simulink model "2_4"  (R2017b)
settings: Solver=FixedStepAuto  StartTime=0.0  StopTime=5  FixedStep=1e-5  MaxStep=1e-4  RelTol=1e-3
libraries: powerlib x25
settings Model: NumberOfSteps=10  Creator=aniko  LastModifiedBy=aniko

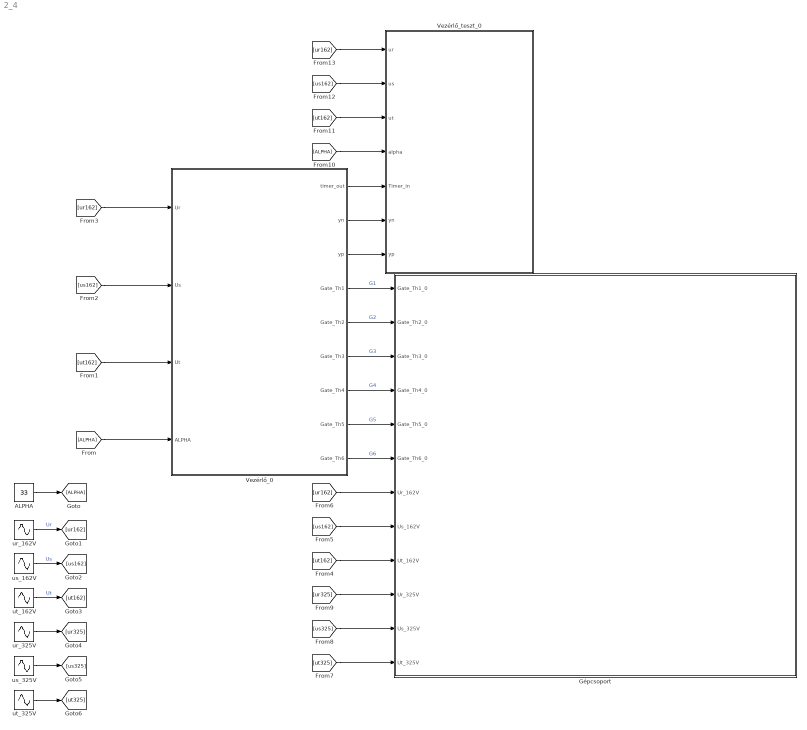
== system 2_4 ==
  "ALPHA " : Constant  Value=33
  "Gépcsoport " : Subsystem
  "Vezérlő_0 " : Subsystem
  Vezérlő_teszt_0 : Subsystem
  ur_162V : Sin  Amplitude=162  Frequency=50*2*pi  Phase=(2/3*pi)+(pi/2)  SampleTime=0
  "ur_325V " : Sin  Amplitude=325  Frequency=50*2*pi  Phase=(2/3*pi)  SampleTime=0
  us_162V : Sin  Amplitude=162  Frequency=50*2*pi  Phase=0+(pi/2)  SampleTime=0
  us_325V : Sin  Amplitude=325  Frequency=50*2*pi  SampleTime=0
  ut_162V : Sin  Amplitude=162  Frequency=50*2*pi  Phase=(4/3*pi)+(pi/2)  SampleTime=0
  ut_325V : Sin  Amplitude=325  Frequency=50*2*pi  Phase=(4/3)*pi  SampleTime=0
  wires:
  "Vezérlő_0 "/9("Gate_Th6 ") -> "Gépcsoport "/6(Gate_Th6_0)  "G6"
  "Vezérlő_0 "/8(Gate_Th5) -> "Gépcsoport "/5(Gate_Th5_0)  "G5"
  "Vezérlő_0 "/7("Gate_Th4 ") -> "Gépcsoport "/4(Gate_Th4_0)  "G4"
  "Vezérlő_0 "/6(Gate_Th3) -> "Gépcsoport "/3(Gate_Th3_0)  "G3"
  "Vezérlő_0 "/5("Gate_Th2 ") -> "Gépcsoport "/2(Gate_Th2_0)  "G2"
  "Vezérlő_0 "/4(Gate_Th1) -> "Gépcsoport "/1("Gate_Th1_0 ")  "G1"
  "ALPHA "/1 -> [ALPHA]
  ur_162V/1 -> [ur162]  "Ur"
  us_162V/1 -> [us162]  "Us"
  ut_162V/1 -> [ut162]  "Ut"
  "ur_325V "/1 -> [ur325]
  us_325V/1 -> [us325]
  ut_325V/1 -> [ut325]
  [ALPHA] -> "Vezérlő_0 "/4(ALPHA)
  [ut162] -> "Vezérlő_0 "/3(Ut)
  [us162] -> "Vezérlő_0 "/2(Us)
  [ur162] -> "Vezérlő_0 "/1(Ur)
  [ur162] -> "Gépcsoport "/7("Ur_162V ")
  [us162] -> "Gépcsoport "/8(Us_162V)
  [ut162] -> "Gépcsoport "/9(Ut_162V)
  [ur325] -> "Gépcsoport "/10(Ur_325V)
  [us325] -> "Gépcsoport "/11(Us_325V)
  [ut325] -> "Gépcsoport "/12("Ut_325V ")
  "Vezérlő_0 "/2(yn) -> Vezérlő_teszt_0/6("yn ")
  "Vezérlő_0 "/3("yp ") -> Vezérlő_teszt_0/7("yp ")
  "Vezérlő_0 "/1(timer_out) -> Vezérlő_teszt_0/5("Timer_in ")
  [ur162] -> Vezérlő_teszt_0/1(ur)
  [us162] -> Vezérlő_teszt_0/2(us)
  [ut162] -> Vezérlő_teszt_0/3("ut ")
  [ALPHA] -> Vezérlő_teszt_0/4("alpha ")

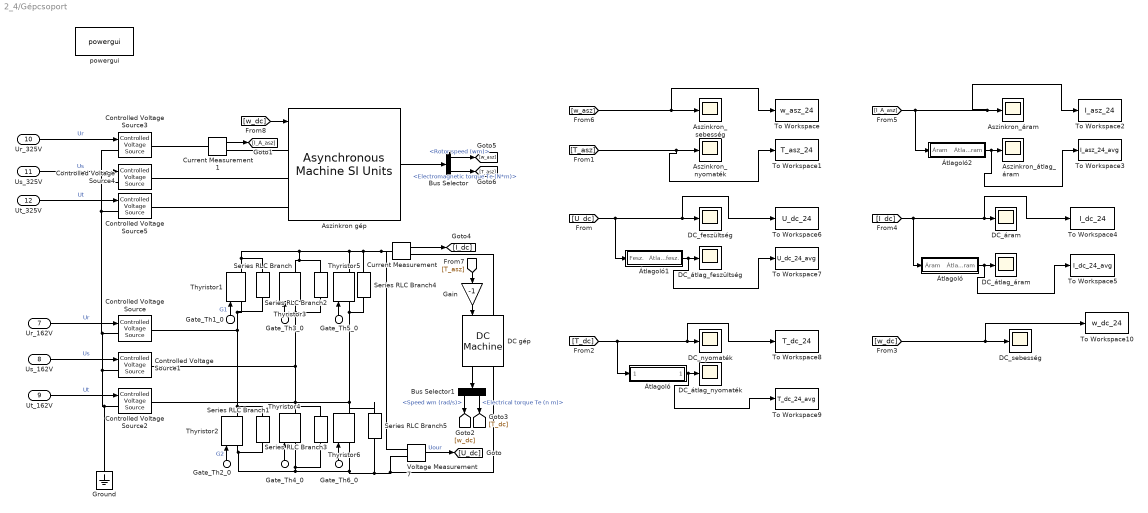
== system 2_4/Gépcsoport  ==
  "Gate_Th1_0 " : Inport
  Gate_Th2_0 : Inport  Port=2
  Gate_Th3_0 : Inport  Port=3
  Gate_Th4_0 : Inport  Port=4
  Gate_Th5_0 : Inport  Port=5
  Gate_Th6_0 : Inport  Port=6
  "Ur_162V " : Inport  Port=7
  Us_162V : Inport  Port=8
  Ut_162V : Inport  Port=9
  Ur_325V : Inport  Port=10
  Us_325V : Inport  Port=11
  "Ut_325V " : Inport  Port=12
  Aszinkron gép : powerlib/Machines/Asynchronous Machine SI Units  RotorType=Squirrel-cage  PresetModel=No  MechanicalLoad=Speed w  ShowDetailedParameters=on  ReferenceFrame=Rotor  Units=SI  MeasurementBus=off  NominalParameters=[5500 400 50]  Stator=[1 0.00565]  Rotor=[1 0.00565]  Cage1=[0.4155 0.002066]  Cage2=[0.4168 0.0003495]  Lm=0.091  Mechanical=[0.05 0.005879 3]  PolePairs=3  InitialConditions=[0 0 0 0 0 0 0 0]  SimulateSaturation=off  Saturation=[14.03593122, 27.81365428, 53.79336849, 72.68890987, 97.98006896, 148.6815601, 215.7428561, 302.9841135, 428.7778367 ; 230, 322, 414, 460, 506, 552, 598, 644, 690]  LoadFlowParameters=1492000  TsPowergui=0  TsBlock=-1  IterativeModel=Trapezoidal non iterative  IterativeDiscreteModel=Trapezoidal non iterative  Pmec=1.492e+006
  "Aszinkron_nyomaték " : Scope
  "Aszinkron_sebesség " : Scope
  Aszinkron_áram : Scope
  Aszinkron_átlag_áram : Scope
  Bus Selector : BusSelector  OutputSignals=Mechanical.Rotor speed (wm),Mechanical.Electromagnetic torque Te (N*m)
  Bus Selector1 : BusSelector  OutputSignals=Speed wm (rad/s),Electrical torque Te (n m)
  Controlled Voltage Source{,1..5} (6 alike) : powerlib/Electrical Sources/Controlled Voltage Source  Initialize=on  Source_Type=AC  Amplitude=0  Phase=0  Frequency=0  Measurements=None
  Current Measurement : powerlib/Measurements/Current Measurement  PhasorSimulation=off  OutputType=Complex  PSBequivalent=0
  Current Measurement1 : powerlib/Measurements/Current Measurement  PhasorSimulation=off  OutputType=Complex  PSBequivalent=0
  DC gép : powerlib/Machines/DC Machine  PresetModel=No  MechanicalLoad=Torque TL  FieldType=Permanent magnet  ShowDetailedParameters=on  MeasurementBus=off  RLa=[ 0.1 10e-3]  RLf="[ 240  120]"  Laf=1.8  MachineConstant=Back-emf constant (V/rpm)  Ke=205/1000  Kt=1.8  J=0.0325  Bm=0  Tf=0  w0=1  Ifinit=1  TsPowergui=0  TsBlock=-1
  "DC_feszültség " : Scope
  "DC_nyomaték " : Scope
  "DC_sebesség " : Scope
  "DC_áram " : Scope
  DC_átlag_feszültség : Scope
  "DC_átlag_nyomaték " : Scope
  DC_átlag_áram : Scope
  Gain : Gain  Gain=-1
  Ground : powerlib/Elements/Ground  LConnTagsString=a
  Series RLC Branch{,1..5} (6 alike) : powerlib/Elements/Series RLC Branch  LConnTagsString=__new0  RConnTagsString=__new0  BranchType=R  Resistance=100000  Inductance=1e-3  SetiL0=off  InitialCurrent=0  Capacitance=1e-6  Setx0=off  InitialVoltage=0  Measurements=None
  Thyristor{1..6} (6 alike) : powerlib/Power Electronics/Thyristor  Ron=0.001  Lon=0  Vf=0.8  IC=0  Rs=inf  Cs=250e-9  Measurements=on
  To Workspace : ToWorkspace  VariableName=w_asz_24  SaveFormat=Timeseries  SampleTime=-1
  To Workspace1 : ToWorkspace  VariableName=T_asz_24  SaveFormat=Timeseries  SampleTime=-1
  To Workspace10 : ToWorkspace  VariableName=w_dc_24  SaveFormat=Timeseries  SampleTime=-1
  To Workspace2 : ToWorkspace  VariableName=I_asz_24  SaveFormat=Timeseries  SampleTime=-1
  To Workspace3 : ToWorkspace  VariableName=I_asz_24_avg  SaveFormat=Timeseries  SampleTime=-1
  To Workspace4 : ToWorkspace  VariableName=I_dc_24  SaveFormat=Timeseries  SampleTime=-1
  To Workspace5 : ToWorkspace  VariableName=I_dc_24_avg  SaveFormat=Timeseries  SampleTime=-1
  To Workspace6 : ToWorkspace  VariableName=U_dc_24  SaveFormat=Timeseries  SampleTime=-1
  To Workspace7 : ToWorkspace  VariableName=U_dc_24_avg  SaveFormat=Timeseries  SampleTime=-1
  To Workspace8 : ToWorkspace  VariableName=T_dc_24  SaveFormat=Timeseries  SampleTime=-1
  To Workspace9 : ToWorkspace  VariableName=T_dc_24_avg  SaveFormat=Timeseries  SampleTime=-1
  Voltage Measurement7 : powerlib/Measurements/Voltage Measurement  PhasorSimulation=off  OutputType=Complex  PSBequivalent=0
  powergui : powerlib/powergui  Priority=1  SimulationMode=Discrete  SampleTime=1e-5  frequency=60  Iterations=50  frequencyindice=0  Pbase=100e6  ErrMax=1e-4  UnitsV=kV  UnitsW=MW  buscounter=0  FunctionMessages=off  echomessages=off  EnableUseOfTLC=off  CurrentSourceSwitches=off  DisableSnubberDevices=off  DisableRonSwitches=off  DisableVfSwitches=off  DisplayEquations=off  SolverType=Tustin/Backward Euler (TBE)  Interpol=off  ExternalGateDelay=off  methode=off  Ts=100  x0status=blocks  SPID=off  SwTol=0  HookPort=off  RestoreLinks=warning  ResistiveCurrentMeasurement=off  Frange=[0:2:500]  Ylog=off  Xlog=on  ShowGrid=off  save=off  variable=ZData  structure=0  ZoomFFT=off  StartTime=0.0  cycles=1  DisplayStyle=1  fundamental=60  FreqAxis=off  MaxFrequency=1000  frequencyindicesteady=1  RmsSteady=1  display=off
  Átlagoló : Subsystem
  "Átlagoló " : Subsystem
  Átlagoló1 : Subsystem
  Átlagoló2 : Subsystem
  wires:
  "Ur_162V "/1 -> Controlled Voltage Source/1  "Ur"
  Us_162V/1 -> Controlled Voltage Source1/1  "Us"
  Ut_162V/1 -> Controlled Voltage Source2/1  "Ut"
  Us_325V/1 -> Controlled Voltage Source4/1  "Us"
  Ur_325V/1 -> Controlled Voltage Source3/1  "Ur"
  "Ut_325V "/1 -> Controlled Voltage Source5/1  "Ut"
  "Gate_Th1_0 "/1 -> Thyristor1/1  "G1"
  Gate_Th3_0/1 -> Thyristor3/1
  Gate_Th4_0/1 -> Thyristor4/1
  Gate_Th5_0/1 -> Thyristor5/1
  Gate_Th6_0/1 -> Thyristor6/1
  Aszinkron gép/1 -> Bus Selector/1
  Voltage Measurement7/1 -> [U_dc]  "Uour"
  Gate_Th2_0/1 -> Thyristor2/1  "G2"
  Gain/1 -> DC gép/1
  Current Measurement1/1 -> [I_A_asz]
  [I_A_asz] -> Átlagoló2/1("Áram "), To Workspace2/1, Aszinkron_áram/1
  Átlagoló/1(Átlag_áram) -> To Workspace5/1, DC_átlag_áram/1
  DC gép/1 -> Bus Selector1/1
  Bus Selector1/1 -> [w_dc]  "<Speed wm (rad/s)>"
  Bus Selector1/2 -> [T_dc]  "<Electrical torque Te (n m)>"
  Átlagoló1/1(Átlag_fesz.) -> To Workspace7/1, DC_átlag_feszültség/1
  [T_dc] -> "Átlagoló "/1("Nyomaték "), To Workspace8/1, "DC_nyomaték "/1
  [w_dc] -> To Workspace10/1, "DC_sebesség "/1
  Current Measurement/1 -> [I_dc]
  [I_dc] -> Átlagoló/1("Áram "), To Workspace4/1, "DC_áram "/1
  Átlagoló2/1(Átlag_áram) -> To Workspace3/1, Aszinkron_átlag_áram/1
  Bus Selector/1 -> [w_asz]  "<Rotor speed (wm)>"
  Bus Selector/2 -> [T_asz]  "<Electromagnetic torque Te (N*m)>"
  [T_asz] -> To Workspace1/1, "Aszinkron_nyomaték "/1
  [w_asz] -> To Workspace/1, "Aszinkron_sebesség "/1
  [T_asz] -> Gain/1
  [w_dc] -> Aszinkron gép/1
  [U_dc] -> Átlagoló1/1("Fesz. "), To Workspace6/1, "DC_feszültség "/1
  "Átlagoló "/1(Átlag_nyomaték) -> To Workspace9/1, "DC_átlag_nyomaték "/1
  connections:
  Series RLC Branch/LConn1 -- Thyristor1/RConn1 -- Thyristor3/RConn1 -- Series RLC Branch2/LConn1 -- Thyristor5/RConn1 -- Current Measurement/LConn1 -- Voltage Measurement7/LConn1 -- Series RLC Branch4/LConn1
  Current Measurement1/LConn1 -- Controlled Voltage Source3/RConn1
  Aszinkron gép/LConn2 -- Controlled Voltage Source4/RConn1
  Aszinkron gép/LConn3 -- Controlled Voltage Source5/RConn1
  Controlled Voltage Source3/LConn1 -- Ground/LConn1 -- Controlled Voltage Source2/LConn1 -- Controlled Voltage Source1/LConn1 -- Controlled Voltage Source/LConn1 -- Controlled Voltage Source5/LConn1 -- Controlled Voltage Source4/LConn1
  Current Measurement1/RConn1 -- Aszinkron gép/LConn1
  Controlled Voltage Source/RConn1 -- Series RLC Branch1/LConn1 -- Thyristor2/RConn1 -- Series RLC Branch/RConn1 -- Thyristor1/LConn1
  Series RLC Branch2/RConn1 -- Thyristor3/LConn1 -- Series RLC Branch3/LConn1 -- Thyristor4/RConn1 -- Controlled Voltage Source1/RConn1
  Controlled Voltage Source2/RConn1 -- Series RLC Branch4/RConn1 -- Thyristor5/LConn1 -- Series RLC Branch5/LConn1 -- Thyristor6/RConn1
  Series RLC Branch1/RConn1 -- Thyristor2/LConn1 -- Thyristor4/LConn1 -- Series RLC Branch3/RConn1 -- DC gép/RConn1 -- Voltage Measurement7/LConn2 -- Series RLC Branch5/RConn1 -- Thyristor6/LConn1
  DC gép/LConn1 -- Current Measurement/RConn1

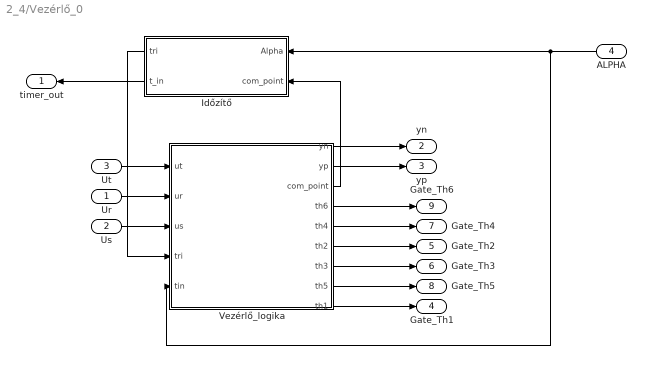
== system 2_4/Vezérlő_0  ==
  Ur : Inport
  Us : Inport  Port=2
  Ut : Inport  Port=3
  ALPHA : Inport  Port=4
  "Időzítő " : Subsystem  TreatAsAtomicUnit=on  SystemSampleTime=1e-5
      settings: MinAlgLoopOccurrences=on
  "Vezérlő_logika " : Stateflow chart  TreatAsAtomicUnit=on
  timer_out : Outport
  yn : Outport  Port=2
  "yp " : Outport  Port=3
  Gate_Th1 : Outport  Port=4
  "Gate_Th2 " : Outport  Port=5
  Gate_Th3 : Outport  Port=6
  "Gate_Th4 " : Outport  Port=7
  Gate_Th5 : Outport  Port=8
  "Gate_Th6 " : Outport  Port=9
  wires:
  Ur/1 -> "Vezérlő_logika "/2(ur)
  Us/1 -> "Vezérlő_logika "/3(us)
  "Vezérlő_logika "/1(yn) -> yn/1
  "Vezérlő_logika "/2(yp) -> "yp "/1
  Ut/1 -> "Vezérlő_logika "/1(ut)
  "Vezérlő_logika "/4(th6) -> "Gate_Th6 "/1
  "Vezérlő_logika "/8(th5) -> Gate_Th5/1
  "Időzítő "/2("t_in ") -> timer_out/1
  "Vezérlő_logika "/5(th4) -> "Gate_Th4 "/1
  "Vezérlő_logika "/7(th3) -> Gate_Th3/1
  "Vezérlő_logika "/9(th1) -> Gate_Th1/1
  "Vezérlő_logika "/6(th2) -> "Gate_Th2 "/1
  "Vezérlő_logika "/3(com_point) -> "Időzítő "/2(com_point)
  "Időzítő "/1(tri) -> "Vezérlő_logika "/4(tri)
  ALPHA/1 -> "Vezérlő_logika "/5(tin), "Időzítő "/1(Alpha)

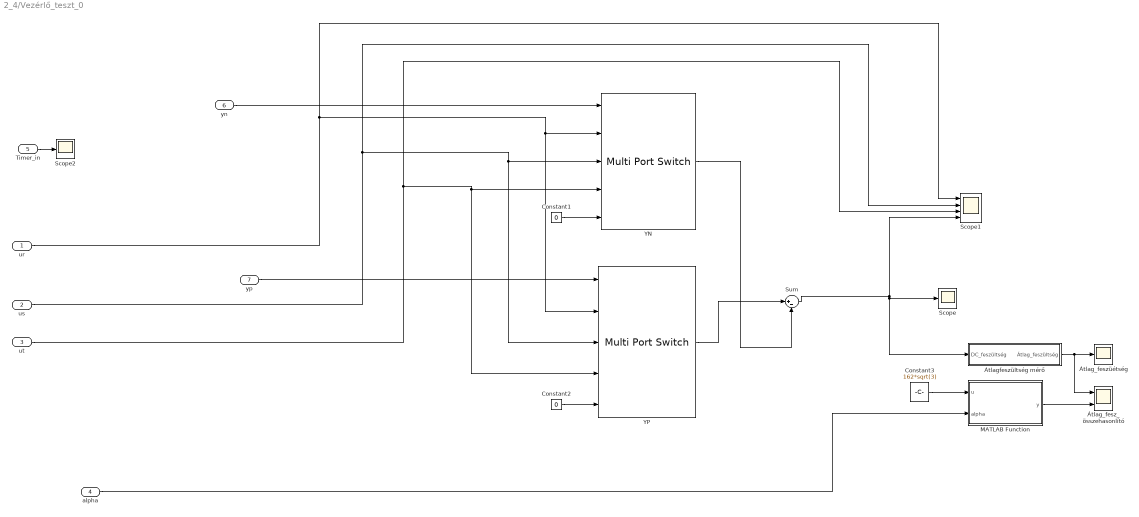
== system 2_4/Vezérlő_teszt_0 ==
  ur : Inport
  us : Inport  Port=2
  "ut " : Inport  Port=3
  "alpha " : Inport  Port=4
  "Timer_in " : Inport  Port=5
  "yn " : Inport  Port=6
  "yp " : Inport  Port=7
  Constant1 : Constant  Value=0
  Constant2 : Constant  Value=0
  Constant3 : Constant  Value=162*sqrt(3)
  MATLAB Function : MATLAB Function  TreatAsAtomicUnit=on
  Scope : Scope
  Scope1 : Scope  NumInputPorts=4
  Scope2 : Scope
  Sum : Sum  Inputs=|+-
  YN : MultiPortSwitch  Inputs=4
  "YP " : MultiPortSwitch  Inputs=4
  "Átlag_fesz_összehasonlító " : Scope  NumInputPorts=2
  "Átlag_feszüétség " : Scope
  Átlagfeszültség mérő : Subsystem
  wires:
  "yp "/1 -> "YP "/1
  "alpha "/1 -> MATLAB Function/2(alpha)
  us/1 -> Scope1/2, "YP "/3, YN/3
  Átlagfeszültség mérő/1("Átlag_feszültség ") -> "Átlag_fesz_összehasonlító "/1, "Átlag_feszüétség "/1
  ur/1 -> Scope1/1, "YP "/2, YN/2
  Constant3/1 -> MATLAB Function/1(u)
  "ut "/1 -> Scope1/3, "YP "/4, YN/4
  Sum/1 -> Scope/1, Átlagfeszültség mérő/1("DC_feszültség "), Scope1/4
  MATLAB Function/1(y) -> "Átlag_fesz_összehasonlító "/2
  Constant1/1 -> YN/5
  "yn "/1 -> YN/1
  Constant2/1 -> "YP "/5
  "Timer_in "/1 -> Scope2/1
  YN/1 -> Sum/2
  "YP "/1 -> Sum/1

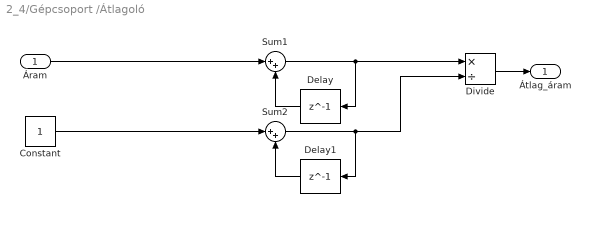
== system 2_4/Gépcsoport /Átlagoló ==
  "Áram " : Inport
  Constant : Constant  SampleTime=-1
  Delay : Delay  DelayLength=1  InitialCondition=0
  Delay1 : Delay  DelayLength=1  InitialCondition=0
  Divide : Product  Inputs=*/
  Sum1 : Sum  Inputs=|++
  Sum2 : Sum  Inputs=|++
  Átlag_áram : Outport
  wires:
  Sum1/1 -> Divide/1, Delay/1
  Delay/1 -> Sum1/2
  "Áram "/1 -> Sum1/1
  Sum2/1 -> Divide/2, Delay1/1
  Delay1/1 -> Sum2/2
  Constant/1 -> Sum2/1
  Divide/1 -> Átlag_áram/1

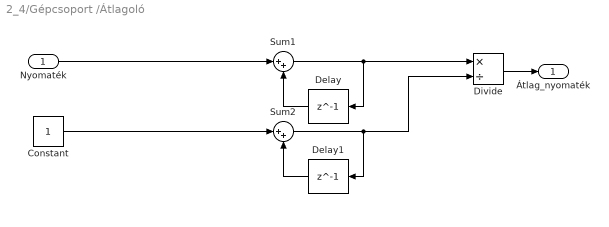
== system 2_4/Gépcsoport /Átlagoló  ==
  "Nyomaték " : Inport
  Constant : Constant  SampleTime=-1
  Delay : Delay  DelayLength=1  InitialCondition=0
  Delay1 : Delay  DelayLength=1  InitialCondition=0
  Divide : Product  Inputs=*/
  Sum1 : Sum  Inputs=|++
  Sum2 : Sum  Inputs=|++
  Átlag_nyomaték : Outport
  wires:
  Sum1/1 -> Divide/1, Delay/1
  Delay/1 -> Sum1/2
  "Nyomaték "/1 -> Sum1/1
  Sum2/1 -> Divide/2, Delay1/1
  Delay1/1 -> Sum2/2
  Constant/1 -> Sum2/1
  Divide/1 -> Átlag_nyomaték/1

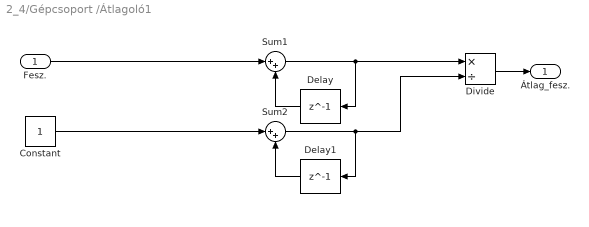
== system 2_4/Gépcsoport /Átlagoló1 ==
  "Fesz. " : Inport
  Constant : Constant  SampleTime=-1
  Delay : Delay  DelayLength=1  InitialCondition=0
  Delay1 : Delay  DelayLength=1  InitialCondition=0
  Divide : Product  Inputs=*/
  Sum1 : Sum  Inputs=|++
  Sum2 : Sum  Inputs=|++
  Átlag_fesz. : Outport
  wires:
  Sum1/1 -> Divide/1, Delay/1
  Delay/1 -> Sum1/2
  "Fesz. "/1 -> Sum1/1
  Sum2/1 -> Divide/2, Delay1/1
  Delay1/1 -> Sum2/2
  Constant/1 -> Sum2/1
  Divide/1 -> Átlag_fesz./1

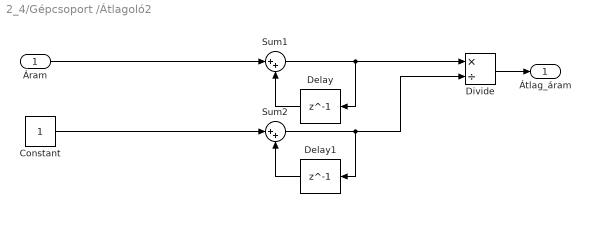
== system 2_4/Gépcsoport /Átlagoló2 ==
  "Áram " : Inport
  Constant : Constant  SampleTime=-1
  Delay : Delay  DelayLength=1  InitialCondition=0
  Delay1 : Delay  DelayLength=1  InitialCondition=0
  Divide : Product  Inputs=*/
  Sum1 : Sum  Inputs=|++
  Sum2 : Sum  Inputs=|++
  Átlag_áram : Outport
  wires:
  Sum1/1 -> Divide/1, Delay/1
  Delay/1 -> Sum1/2
  "Áram "/1 -> Sum1/1
  Sum2/1 -> Divide/2, Delay1/1
  Delay1/1 -> Sum2/2
  Constant/1 -> Sum2/1
  Divide/1 -> Átlag_áram/1

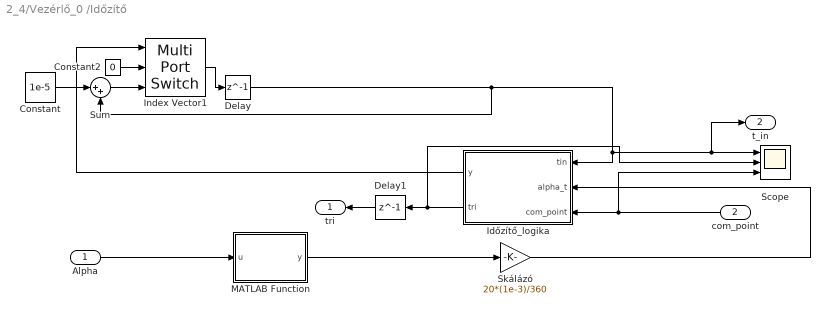
== system 2_4/Vezérlő_0 /Időzítő  ==
  Alpha : Inport
  com_point : Inport  Port=2
  Constant : Constant  Value=1e-5  SampleTime=-1
  Constant2 : Constant  Value=0
  Delay : Delay  DelayLength=1  InitialCondition=0
  Delay1 : Delay  DelayLength=1  InitialCondition=0
  "Időzítő_logika " : Stateflow chart  TreatAsAtomicUnit=on
  Index Vector1 : MultiPortSwitch  DataPortOrder=Zero-based contiguous  Inputs=2  zeroidx=on
  MATLAB Function : MATLAB Function  TreatAsAtomicUnit=on
  Scope : Scope  NumInputPorts=3
  Skálázó : Gain  Gain=20*(1e-3)/360
  Sum : Sum  Inputs=|++
  tri : Outport
  "t_in " : Outport  Port=2
  wires:
  Sum/1 -> Index Vector1/3
  Constant/1 -> Sum/1
  "Időzítő_logika "/1(y) -> Index Vector1/1
  Skálázó/1 -> "Időzítő_logika "/2(alpha_t)
  com_point/1 -> Scope/3, "Időzítő_logika "/3(com_point)
  "Időzítő_logika "/2(tri) -> Delay1/1, Scope/2
  Delay/1 -> "Időzítő_logika "/1(tin), "t_in "/1, Scope/1, Sum/2
  Constant2/1 -> Index Vector1/2
  Index Vector1/1 -> Delay/1
  Delay1/1 -> tri/1
  MATLAB Function/1(y) -> Skálázó/1
  Alpha/1 -> MATLAB Function/1(u)

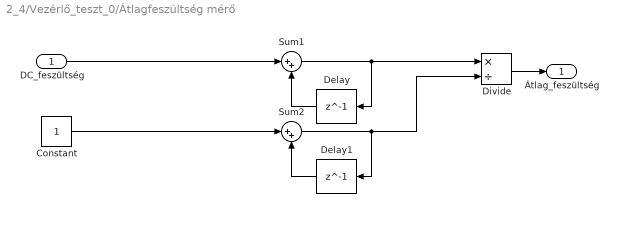
== system 2_4/Vezérlő_teszt_0/Átlagfeszültség mérő ==
  "DC_feszültség " : Inport
  Constant : Constant  SampleTime=-1
  Delay : Delay  DelayLength=1  InitialCondition=0
  Delay1 : Delay  DelayLength=1  InitialCondition=0
  Divide : Product  Inputs=*/
  Sum1 : Sum  Inputs=|++
  Sum2 : Sum  Inputs=|++
  "Átlag_feszültség " : Outport
  wires:
  Sum1/1 -> Divide/1, Delay/1
  Delay/1 -> Sum1/2
  "DC_feszültség "/1 -> Sum1/1
  Sum2/1 -> Divide/2, Delay1/1
  Delay1/1 -> Sum2/2
  Constant/1 -> Sum2/1
  Divide/1 -> "Átlag_feszültség "/1

== matlab function 2_4/Vezérlő_teszt_0/MATLAB Function ==
  data: u input; y output; alpha input
function y =aramiranyito(u, alpha)

%Az áramirányító elméleti kimeneti feszültsége.

y=u*(3/pi)*cos((alpha*(2*pi)/360));

== matlab function 2_4/Vezérlő_0 /Időzítő /MATLAB Function ==
  data: u input; y output
function y =idozito(u)
%Az időzítő helyes beállítására szolgál.


if u<=0,
 y=0;
elseif u>0 && u<60,
 y=u;
elseif u>=60 && u<120,
 y=u-60;    
elseif u>=120 && u<180,
 y=u-120;
else
 y=59;
end;

== stateflow chart 2_4/Vezérlő_0 /Időzítő /Időzítő_logika  ==
  state RESET
    during: y=0;
    tri=0;
  state COUNTING
    during: y=1;
    tri=0;
  state Trans
    during: y=0;
    tri=0;
  state TRIGGER
    during:
    y=1;
    tri=1;
  (default) -> RESET
  RESET -> COUNTING : [com_point==1]
  Trans -> COUNTING : [com_point==1]
  COUNTING -> TRIGGER : [tin>=alpha_t]
  TRIGGER -> Trans : [com_point==0]
  data: y output; tin input; alpha_t input; com_point input; tri output

== stateflow chart 2_4/Vezérlő_0 /Vezérlő_logika  ==
  state GY36_120
    entry:
    com_point=0;
    th1=0;
    th2=0;
    th3=1
    th4=0;
    th5=0;
    th6=1;
    yp=2;
    yn=3;
  state GY16_120
    entry:
    com_point=0;
    th1=1;
    th2=0;
    th3=0;
    th4=0;
    th5=0;
    th6=1;
    yp=1;
    yn=3;
  state GY54_120
    entry:
    com_point=0;
    th1=0;
    th2=0;
    th3=0;
    th4=1;
    th5=1;
    th6=0;
    yp=3;
    yn=2;
  state GY14_120
    entry:
    com_point=0;
    th1=1;
    th2=0;
    th3=0;
    th4=1;
    th5=0;
    th6=0;
    yp=1;
    yn=2;
  state GY32_120
    entry:
    com_point=0;
    th1=0;
    th2=1;
    th3=1;
    th4=0;
    th5=0;
    th6=0;
    yp=2;
    yn=1;
  state GY52_120
    entry:
    com_point=0;
    th1=0;
    th2=1;
    th3=0;
    th4=0;
    th5=1;
    th6=0;
    yp=3;
    yn=1;
  state utmax_urmin_120
    entry:
    com_point=1;
  state utmax_usmin_120
    entry:
    com_point=1;
  state usmax_urmin_120
    entry:
    com_point=1;
  state urmax_usmin_120
    entry:
    com_point=1;
  state urmax_utmin_120
    entry:
    com_point=1;
  state usmax_utmin_120
    entry:
    com_point=1;
  state START
    entry: yp=4;
    yn=4;
    com_point=0;
    th1=0;
    th2=0;
    th3=0;
    th4=0;
    th5=0;
    th6=0;
  state urmax_utmin_60
    entry:
    com_point=1;
  state usmax_utmin_60
    entry:
    com_point=1;
  state utmax_urmin_60
    entry:
    com_point=1;
  state utmax_usmin_60
    entry:
    com_point=1;
  state usmax_urmin_60
    entry:
    com_point=1;
  state urmax_usmin_60
    entry:
    com_point=1;
  state urmax_utmin_0
    entry:
    com_point=1;
  state usmax_utmin_0
    entry:
    com_point=1;
  state utmax_urmin_0
    entry:
    com_point=1;
  state utmax_usmin_0
    entry:
    com_point=1;
  state usmax_urmin_0
    entry:
    com_point=1;
  state urmax_usmin_0
    entry:
    com_point=1;
  state GY16_60
    entry:
    com_point=0;
    th1=1;
    th2=0;
    th3=0;
    th4=0;
    th5=0;
    th6=1;
    yp=1;
    yn=3;
  state GY14_60
    entry:
    com_point=0;
    th1=1;
    th2=0;
    th3=0;
    th4=1;
    th5=0;
    th6=0;
    yp=1;
    yn=2;
  state GY36_60
    entry:
    com_point=0;
    th1=0;
    th2=0;
    th3=1;
    th4=0;
    th5=0;
    th6=1;
    yp=2;
    yn=3;
  state GY54_60
    entry:
    com_point=0;
    th1=0;
    th2=0;
    th3=0;
    th4=1;
    th5=1;
    th6=0;
    yp=3;
    yn=2;
  state GY32_60
    entry:
    com_point=0;
    th1=0;
    th2=1;
    th3=1;
    th4=0;
    th5=0;
    th6=0;
    yp=2;
    yn=1;
  state GY52_60
    entry:
    com_point=0;
    th1=0;
    th2=1;
    th3=0;
    th4=0;
    th5=1;
    th6=0;
    yp=3;
    yn=1;
  state GY16_0
    entry:
    com_point=0;
    th1=1;
    th2=0;
    th3=0;
    th4=0;
    th5=0;
    th6=1;
    yp=1;
    yn=3;
  state GY32_0
    entry:
    com_point=0;
    th1=0;
    th2=1;
    th3=1;
    th4=0;
    th5=0;
    th6=0;
    yp=2;
    yn=1;
  state GY14_0
    entry:
    com_point=0;
    th1=1;
    th2=0;
    th3=0;
    th4=1;
    th5=0;
    th6=0;
    yp=1;
    yn=2;
  state GY54_0
    entry:
    com_point=0;
    th1=0;
    th2=0;
    th3=0;
    th4=1;
    th5=1;
    th6=0;
    yp=3;
    yn=2;
  state GY36_0
    entry:
    com_point=0;
    th1=0;
    th2=0;
    th3=1;
    th4=0;
    th5=0;
    th6=1;
    yp=2;
    yn=3;
  state GY52_0
    entry:
    com_point=0;
    th1=0;
    th2=1;
    th3=0;
    th4=0;
    th5=1;
    th6=0;
    yp=3;
    yn=1;
  GY32_120 -> urmax_usmin_120 : [ur>ut &&us<ut]
  GY16_120 -> utmax_urmin_120 : [ut>us && ur<us]
  GY54_120 -> usmax_utmin_120 : [us>ur && ut<ur]
  GY14_120 -> usmax_urmin_120 : [us>ut && ur<ut]
  GY36_120 -> utmax_usmin_120 : [ut>ur && us<ur]
  GY52_120 -> urmax_utmin_120 : [ur>us && ut<us]
  utmax_urmin_120 -> GY36_120 [order 2] : [tri==1]
  urmax_utmin_120 -> GY54_120 [order 2] : [tri==1]
  utmax_usmin_120 -> GY32_120 [order 1] : [tri==1]
  usmax_utmin_120 -> GY14_120 [order 2] : [tri==1]
  usmax_urmin_120 -> GY16_120 [order 2] : [tri==1]
  urmax_usmin_120 -> GY52_120 [order 2] : [tri==1]
  usmax_urmin_120 -> utmax_urmin_120 [order 1] : [ut>us && ur<us]
  usmax_utmin_120 -> usmax_urmin_120 [order 1] : [us>ut && ur<ut]
  utmax_urmin_120 -> utmax_usmin_120 [order 1] : [ut>ur && us<ur]
  START -> utmax_usmin_60 [order 2] : [ut>ur&& us<ur && 60<=tin && tin<120]
  urmax_usmin_120 -> urmax_utmin_120 [order 1] : [ur>us && ut<us]
  urmax_utmin_120 -> usmax_utmin_120 [order 1] : [us>ur && ut<ur]
  START -> utmax_urmin_60 [order 12] : [ut>us &&ur<us&&60<=tin&&tin<120]
  utmax_usmin_120 -> urmax_usmin_120 [order 2] : [ur>ut && us<ut]
  START -> utmax_urmin_120 [order 17] : [ut>us&&ur<us&&tin>=120]
  START -> urmax_usmin_120 [order 13] : [ur>ut &&us<ut&&tin>=120]
  START -> urmax_utmin_120 [order 14] : [ur>us&&ut<us&&tin>=120]
  START -> usmax_utmin_120 [order 15] : [us>ur&&ut<ur&&tin>=120]
  START -> usmax_urmin_60 [order 11] : [us>ut&&ur<ut&& 60<=tin && tin<120]
  START -> usmax_urmin_120 [order 16] : [us>ut&&ur<ut&&tin>=120]
  START -> utmax_usmin_120 [order 18] : [ut>ur&&us<ur&&tin>=120]
  START -> usmax_utmin_60 [order 10] : [us>ur&&ut<ur&& 60<=tin && tin<120]
  START -> urmax_utmin_60 [order 9] : [ur>us && ut<us && 60<=tin && tin<120]
  START -> urmax_usmin_60 [order 8] : [ur>ut && us<ut && 60<=tin && tin<120]
  (default) -> START
  utmax_urmin_60 -> utmax_usmin_60 [order 1] : [ut>ur && us<ur]
  usmax_utmin_60 -> usmax_urmin_60 [order 1] : [us>ut && ur<ut]
  usmax_urmin_60 -> utmax_urmin_60 [order 1] : [ut>us && ur<us]
  urmax_utmin_60 -> usmax_utmin_60 [order 1] : [us>ur && ut<ur]
  urmax_usmin_60 -> urmax_utmin_60 [order 1] : [ur>us && ut<us]
  START -> urmax_usmin_0 [order 3] : [ur>ut &&us<ut&&tin<60]
  START -> urmax_utmin_0 [order 4] : [ur>us &&ut<us&&tin<60]
  START -> usmax_utmin_0 [order 5] : [us>ur &&ut<ur&&tin<60]
  START -> usmax_urmin_0 [order 1] : [us>ut &&ur<ut&&tin<60]
  START -> utmax_urmin_0 [order 6] : [ut>us &&ur<us&&tin<60]
  START -> utmax_usmin_0 [order 7] : [ut>ur &&us<ur&&tin<60]
  utmax_usmin_60 -> urmax_usmin_60 [order 2] : [ur>ut && us<ut]
  GY52_60 -> urmax_usmin_60 : [ur>ut &&us<ut]
  GY54_60 -> urmax_utmin_60 : [ur>us && ut<us]
  urmax_utmin_60 -> GY14_60 [order 2] : [tri==1]
  GY14_60 -> usmax_utmin_60 : [us>ur && ut<ur]
  usmax_utmin_60 -> GY16_60 [order 2] : [tri==1]
  GY16_60 -> usmax_urmin_60 : [us>ut && ur<ut]
  usmax_urmin_60 -> GY36_60 [order 2] : [tri==1]
  GY32_60 -> utmax_usmin_60 : [ut>ur && us<ur]
  utmax_usmin_60 -> GY52_60 [order 1] : [tri==1]
  GY36_60 -> utmax_urmin_60 : [ut>us && ur<us]
  utmax_urmin_60 -> GY32_60 [order 2] : [tri==1]
  urmax_usmin_60 -> GY54_60 [order 2] : [tri==1]
  utmax_urmin_0 -> utmax_usmin_0 [order 1] : [ut>ur && us<ur]
  usmax_utmin_0 -> usmax_urmin_0 [order 1] : [us>ut && ur<ut]
  usmax_urmin_0 -> utmax_urmin_0 [order 1] : [ut>us && ur<us]
  urmax_utmin_0 -> usmax_utmin_0 [order 1] : [us>ur && ut<ur]
  urmax_usmin_0 -> urmax_utmin_0 [order 1] : [ur>us && ut<us]
  utmax_usmin_0 -> urmax_usmin_0 [order 2] : [ur>ut && us<ut]
  GY54_0 -> urmax_usmin_0 : [ur>ut &&us<ut]
  GY14_0 -> urmax_utmin_0 : [ur>us && ut<us]
  urmax_utmin_0 -> GY16_0 [order 2] : [tri==1]
  GY16_0 -> usmax_utmin_0 : [us>ur && ut<ur]
  usmax_utmin_0 -> GY36_0 [order 2] : [tri==1]
  GY36_0 -> usmax_urmin_0 : [us>ut && ur<ut]
  usmax_urmin_0 -> GY32_0 [order 2] : [tri==1]
  GY52_0 -> utmax_usmin_0 : [ut>ur && us<ur]
  utmax_usmin_0 -> GY54_0 [order 1] : [tri==1]
  GY32_0 -> utmax_urmin_0 : [ut>us && ur<us]
  utmax_urmin_0 -> GY52_0 [order 2] : [tri==1]
  urmax_usmin_0 -> GY14_0 [order 2] : [tri==1]
  data: ut input; ur input; us input; yn output; yp output; tri input; com_point output; th6 output; th4 output; th2 output; th3 output; th5 output; th1 output; tin input
